simulink model "steamjacket_test2020b"  (R2020b)
settings: Solver=VariableStepAuto  StartTime=0.0  StopTime=10.0  RelTol=1e-3
settings Model: Creator=Adam  LastModifiedBy=Adam

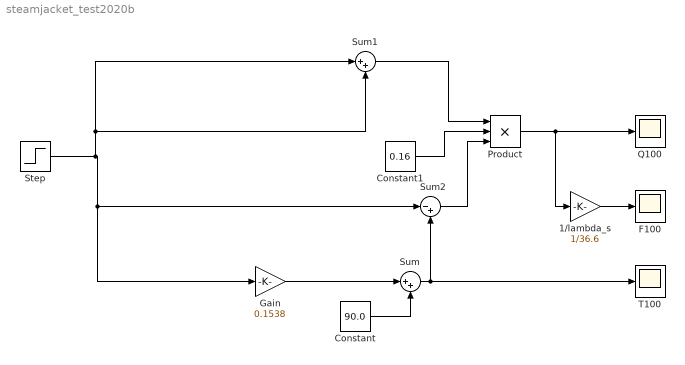
== system steamjacket_test2020b ==
  1/lambda_s : Gain  Gain=1/36.6
  Constant : Constant  Value=90.0
  Constant1 : Constant  Value=0.16
  F100 : Scope
  Gain : Gain  Gain=0.1538
  Product : Product  Inputs=3
  Q100 : Scope
  Step : Step  SampleTime=0
  Sum : Sum  Inputs=|++
  Sum1 : Sum  Inputs=|++
  Sum2 : Sum  Inputs=|-+
  T100 : Scope
  wires:
  Constant/1 -> Sum/2
  Step/1 -> Sum1/2, Sum1/1, Gain/1, Sum2/1
  Gain/1 -> Sum/1
  Sum/1 -> T100/1, Sum2/2
  Sum1/1 -> Product/1
  Constant1/1 -> Product/2
  Sum2/1 -> Product/3
  Product/1 -> Q100/1, 1/lambda_s/1
  1/lambda_s/1 -> F100/1
